simulink model "MOSSE_HDL_final"  (Simulink 8.3)
settings: Solver=FixedStepDiscrete  SolverMode=SingleTasking  StartTime=0.0  StopTime=30*640*360  RelTol=1e-3
InitFcn:
  | %% DSPBuilder Start
  | alt_dspbuilder_update_model(bdroot)
  | %% DSPBuilder End
  | param
StopFcn:
  | % r = rcount.Data(:,:);
  | % w = wcount.Data(:,:);
  | % d = dout.Data(:,:);
  | % ir = read.Data(:,:);
  | % iw = write.Data(:,:);
  | % z = double([ir iw d r w]');
  | %logic_analyzer
values from neighbouring files (symbols this model uses):
  Gau = [4035 -3983 3832 -3589 3269 -2890 2472 -2039 1612 -1211 854 -553 ... (4096 elements, 1x4096)]    [Gauss_coeff.mat]    (also in param.m = reshape(conj(Gau'), 1, 4096))
undefined symbols (not defined in the file or in its folder): gray, psr, source_1, source_2, State_Machine, State_Transition_Table1, window_hann
libraries: allblocks_alteradspbuilder2 x166, hdlsllib x24, hdldemolib x3, simulink x2, dspsigattribs x2, dspmtrx3 x2, visionsinks x1, visiontextngfix x1, dspvision x1
(part 2 of 4)

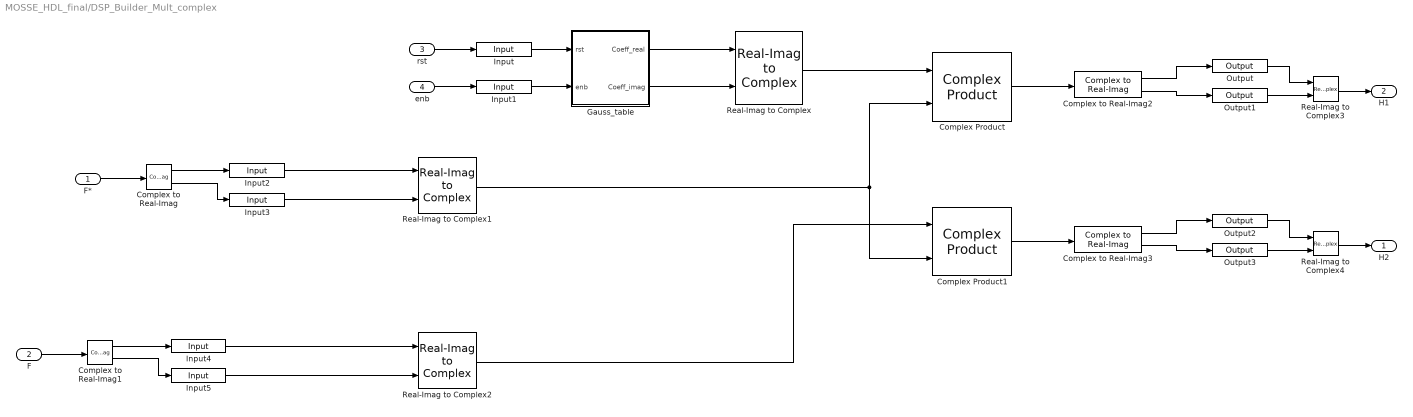
== system MOSSE_HDL_final/DSP_Builder_Mult_complex ==
  F* : Inport
  F : Inport  Port=2
  rst : Inport  Port=3
  enb : Inport  Port=4
  Complex Product : allblocks_alteradspbuilder2/Complex Product  BusType=Inferred  bwl=8  bwr=0  pipeline_register=Multiplier Only  pipeline_display=1  use_ena=off  use_aclr=off  UseDedicatedCircuitry=off  allowFloatingPointOverride=on  logOutputs=off  logFile=E:\Work\ComputerVision\ObjectTrack\MOSSE\autotrackigproject\Model\MOSSE_algorithm\MOSSE_simulink\tb_MOSSE_HDL_final\MOSSE%5FHDL%5Ffinal_DSP%5FBuilder%5FMult%5Fcomplex_Complex+Product.fixedpointlog
  Complex Product1 : allblocks_alteradspbuilder2/Complex Product  BusType=Inferred  bwl=8  bwr=0  pipeline_register=Multiplier Only  pipeline_display=1  use_ena=off  use_aclr=off  UseDedicatedCircuitry=off  allowFloatingPointOverride=on  logOutputs=off  logFile=E:\Work\ComputerVision\ObjectTrack\MOSSE\autotrackigproject\Model\MOSSE_algorithm\MOSSE_simulink\tb_MOSSE_HDL_final\MOSSE%5FHDL%5Ffinal_DSP%5FBuilder%5FMult%5Fcomplex_Complex+Product1.fixedpointlog
  Complex to Real-Imag : ComplexToRealImag
  Complex to Real-Imag1 : ComplexToRealImag
  Complex to Real-Imag2 : allblocks_alteradspbuilder2/Complex to Real-Imag  BusType=Signed Integer  bwl=32  bwr=0  pipeline_display=0  allowFloatingPointOverride=on  logOutputs=off  logFile=E:\Work\ComputerVision\ObjectTrack\MOSSE\autotrackigproject\Model\MOSSE_algorithm\MOSSE_simulink\tb_MOSSE_HDL_final\MOSSE%5FHDL%5Ffinal_DSP%5FBuilder%5FMult%5Fcomplex_Complex+to+Real-Imag2%3A%3Aoutput%5Freal.fixedpointlog,E:\Work\ComputerVision\ObjectTrack\MOSSE\autotrackigproject\Model\MOSSE_algorithm\MOSSE_simulink\tb_MOSSE_HDL_final\MOSSE%5FHDL%5Ffinal_DSP%5FBuilder%5FMult%5Fcomplex_Complex+to+Real-Imag2%3A%3Aoutput%5Fimag.fixedpointlog,
  Complex to Real-Imag3 : allblocks_alteradspbuilder2/Complex to Real-Imag  BusType=Signed Integer  bwl=32  bwr=0  pipeline_display=0  allowFloatingPointOverride=on  logOutputs=off  logFile=E:\Work\ComputerVision\ObjectTrack\MOSSE\autotrackigproject\Model\MOSSE_algorithm\MOSSE_simulink\tb_MOSSE_HDL_final\MOSSE%5FHDL%5Ffinal_DSP%5FBuilder%5FMult%5Fcomplex_Complex+to+Real-Imag3%3A%3Aoutput%5Freal.fixedpointlog,E:\Work\ComputerVision\ObjectTrack\MOSSE\autotrackigproject\Model\MOSSE_algorithm\MOSSE_simulink\tb_MOSSE_HDL_final\MOSSE%5FHDL%5Ffinal_DSP%5FBuilder%5FMult%5Fcomplex_Complex+to+Real-Imag3%3A%3Aoutput%5Fimag.fixedpointlog,
  Gauss_table : Subsystem
  Input : allblocks_alteradspbuilder2/Input  iofile=E:\Work\ComputerVision\ObjectTrack\MOSSE\autotrackigproject\Model\MOSSE_algorithm\MOSSE_simulink\tb_MOSSE_HDL_final\MOSSE%5FHDL%5Ffinal_DSP%5FBuilder%5FMult%5Fcomplex_Input.salt  BusType=Single Bit  bwl=8  bwr=0  SpecifyClock=off  PORTTYPE=Input  externalType=Inferred  allowFloatingPointOverride=on  logOutputs=off
  Input1 : allblocks_alteradspbuilder2/Input  iofile=E:\Work\ComputerVision\ObjectTrack\MOSSE\autotrackigproject\Model\MOSSE_algorithm\MOSSE_simulink\tb_MOSSE_HDL_final\MOSSE%5FHDL%5Ffinal_DSP%5FBuilder%5FMult%5Fcomplex_Input1.salt  BusType=Single Bit  bwl=8  bwr=0  SpecifyClock=off  PORTTYPE=Input  externalType=Inferred  allowFloatingPointOverride=on  logOutputs=off
  Input2 : allblocks_alteradspbuilder2/Input  iofile=E:\Work\ComputerVision\ObjectTrack\MOSSE\autotrackigproject\Model\MOSSE_algorithm\MOSSE_simulink\tb_MOSSE_HDL_final\MOSSE%5FHDL%5Ffinal_DSP%5FBuilder%5FMult%5Fcomplex_Input2.salt  BusType=Signed Integer  bwl=32  bwr=0  SpecifyClock=off  PORTTYPE=Input  externalType=Inferred  allowFloatingPointOverride=on  logOutputs=off
  Input3 : allblocks_alteradspbuilder2/Input  iofile=E:\Work\ComputerVision\ObjectTrack\MOSSE\autotrackigproject\Model\MOSSE_algorithm\MOSSE_simulink\tb_MOSSE_HDL_final\MOSSE%5FHDL%5Ffinal_DSP%5FBuilder%5FMult%5Fcomplex_Input3.salt  BusType=Signed Integer  bwl=32  bwr=0  SpecifyClock=off  PORTTYPE=Input  externalType=Inferred  allowFloatingPointOverride=on  logOutputs=off
  Input4 : allblocks_alteradspbuilder2/Input  iofile=E:\Work\ComputerVision\ObjectTrack\MOSSE\autotrackigproject\Model\MOSSE_algorithm\MOSSE_simulink\tb_MOSSE_HDL_final\MOSSE%5FHDL%5Ffinal_DSP%5FBuilder%5FMult%5Fcomplex_Input4.salt  BusType=Signed Integer  bwl=32  bwr=0  SpecifyClock=off  PORTTYPE=Input  externalType=Inferred  allowFloatingPointOverride=on  logOutputs=off
  Input5 : allblocks_alteradspbuilder2/Input  iofile=E:\Work\ComputerVision\ObjectTrack\MOSSE\autotrackigproject\Model\MOSSE_algorithm\MOSSE_simulink\tb_MOSSE_HDL_final\MOSSE%5FHDL%5Ffinal_DSP%5FBuilder%5FMult%5Fcomplex_Input5.salt  BusType=Signed Integer  bwl=32  bwr=0  SpecifyClock=off  PORTTYPE=Input  externalType=Inferred  allowFloatingPointOverride=on  logOutputs=off
  Output : allblocks_alteradspbuilder2/Output  iofile=E:\Work\ComputerVision\ObjectTrack\MOSSE\autotrackigproject\Model\MOSSE_algorithm\MOSSE_simulink\tb_MOSSE_HDL_final\MOSSE%5FHDL%5Ffinal_DSP%5FBuilder%5FMult%5Fcomplex_Output.capture  BusType=Signed Integer  bwl=32  bwr=0  externalType=Inferred  PORTTYPE=Output  allowFloatingPointOverride=on  logOutputs=off
  Output1 : allblocks_alteradspbuilder2/Output  iofile=E:\Work\ComputerVision\ObjectTrack\MOSSE\autotrackigproject\Model\MOSSE_algorithm\MOSSE_simulink\tb_MOSSE_HDL_final\MOSSE%5FHDL%5Ffinal_DSP%5FBuilder%5FMult%5Fcomplex_Output1.capture  BusType=Signed Integer  bwl=32  bwr=0  externalType=Simulink Fixed Point Type  PORTTYPE=Output  allowFloatingPointOverride=on  logOutputs=off
  Output2 : allblocks_alteradspbuilder2/Output  iofile=E:\Work\ComputerVision\ObjectTrack\MOSSE\autotrackigproject\Model\MOSSE_algorithm\MOSSE_simulink\tb_MOSSE_HDL_final\MOSSE%5FHDL%5Ffinal_DSP%5FBuilder%5FMult%5Fcomplex_Output2.capture  BusType=Signed Integer  bwl=32  bwr=0  externalType=Simulink Fixed Point Type  PORTTYPE=Output  allowFloatingPointOverride=on  logOutputs=off
  Output3 : allblocks_alteradspbuilder2/Output  iofile=E:\Work\ComputerVision\ObjectTrack\MOSSE\autotrackigproject\Model\MOSSE_algorithm\MOSSE_simulink\tb_MOSSE_HDL_final\MOSSE%5FHDL%5Ffinal_DSP%5FBuilder%5FMult%5Fcomplex_Output3.capture  BusType=Signed Integer  bwl=32  bwr=0  externalType=Simulink Fixed Point Type  PORTTYPE=Output  allowFloatingPointOverride=on  logOutputs=off
  Real-Imag to Complex3 : RealImagToComplex
  Real-Imag to Complex4 : RealImagToComplex
  Real-Imag to Complex : allblocks_alteradspbuilder2/Real-Imag to Complex  BusType=Signed Integer  bwl=16  bwr=0  pipeline_display=0  allowFloatingPointOverride=on  logOutputs=off  logFile=E:\Work\ComputerVision\ObjectTrack\MOSSE\autotrackigproject\Model\MOSSE_algorithm\MOSSE_simulink\tb_MOSSE_HDL_final\MOSSE%5FHDL%5Ffinal_DSP%5FBuilder%5FMult%5Fcomplex_Real-Imag+to+Complex.fixedpointlog
  Real-Imag to Complex1 : allblocks_alteradspbuilder2/Real-Imag to Complex  BusType=Signed Integer  bwl=32  bwr=0  pipeline_display=0  allowFloatingPointOverride=on  logOutputs=off  logFile=E:\Work\ComputerVision\ObjectTrack\MOSSE\autotrackigproject\Model\MOSSE_algorithm\MOSSE_simulink\tb_MOSSE_HDL_final\MOSSE%5FHDL%5Ffinal_DSP%5FBuilder%5FMult%5Fcomplex_Real-Imag+to+Complex1.fixedpointlog
  Real-Imag to Complex2 : allblocks_alteradspbuilder2/Real-Imag to Complex  BusType=Signed Integer  bwl=32  bwr=0  pipeline_display=0  allowFloatingPointOverride=on  logOutputs=off  logFile=E:\Work\ComputerVision\ObjectTrack\MOSSE\autotrackigproject\Model\MOSSE_algorithm\MOSSE_simulink\tb_MOSSE_HDL_final\MOSSE%5FHDL%5Ffinal_DSP%5FBuilder%5FMult%5Fcomplex_Real-Imag+to+Complex2.fixedpointlog
  H2 : Outport
  H1 : Outport  Port=2
  wires:
  Gauss_table/1(Coeff_real) -> Real-Imag to Complex/1
  Gauss_table/2(Coeff_imag) -> Real-Imag to Complex/2
  Real-Imag to Complex/1 -> Complex Product/1
  rst/1 -> Input/1
  Input/1 -> Gauss_table/1(rst)
  enb/1 -> Input1/1
  Input1/1 -> Gauss_table/2(enb)
  F*/1 -> Complex to Real-Imag/1
  F/1 -> Complex to Real-Imag1/1
  Complex to Real-Imag/1 -> Input2/1
  Complex to Real-Imag/2 -> Input3/1
  Complex to Real-Imag1/1 -> Input4/1
  Complex to Real-Imag1/2 -> Input5/1
  Input2/1 -> Real-Imag to Complex1/1
  Input3/1 -> Real-Imag to Complex1/2
  Input4/1 -> Real-Imag to Complex2/1
  Input5/1 -> Real-Imag to Complex2/2
  Real-Imag to Complex1/1 -> Complex Product1/2, Complex Product/2
  Real-Imag to Complex2/1 -> Complex Product1/1
  Complex Product/1 -> Complex to Real-Imag2/1
  Complex to Real-Imag2/2 -> Output1/1
  Complex to Real-Imag2/1 -> Output/1
  Real-Imag to Complex3/1 -> H1/1
  Output/1 -> Real-Imag to Complex3/1
  Output1/1 -> Real-Imag to Complex3/2
  Complex Product1/1 -> Complex to Real-Imag3/1
  Complex to Real-Imag3/2 -> Output3/1
  Complex to Real-Imag3/1 -> Output2/1
  Real-Imag to Complex4/1 -> H2/1
  Output2/1 -> Real-Imag to Complex4/1
  Output3/1 -> Real-Imag to Complex4/2

== system MOSSE_HDL_final/DSP_Builder_PSR ==
  max : Inport
  mean : Inport  Port=2
  tmp : Inport  Port=3
  psr_reset : Inport  Port=4
  Comparator : allblocks_alteradspbuilder2/Comparator  direction=a > b  pipeline_display=0  allowFloatingPointOverride=on  logOutputs=off  logFile=E:\Work\ComputerVision\ObjectTrack\MOSSE\autotrackigproject\Model\MOSSE_algorithm\MOSSE_simulink\tb_MOSSE_HDL_final\MOSSE%5FHDL%5Ffinal_DSP%5FBuilder%5FPSR_Comparator.fixedpointlog
  Constant : allblocks_alteradspbuilder2/Constant  mask_cst=PSR  BusType=Signed Integer  bwl=16  bwr=0  roundMode=Truncate  satMode=Wrap  SpecifyClock=off  allowFloatingPointOverride=on  logOutputs=off  logFile=E:\Work\ComputerVision\ObjectTrack\MOSSE\autotrackigproject\Model\MOSSE_algorithm\MOSSE_simulink\tb_MOSSE_HDL_final\MOSSE%5FHDL%5Ffinal_DSP%5FBuilder%5FPSR_Constant.fixedpointlog
  Data : allblocks_alteradspbuilder2/Input  iofile=E:\Work\ComputerVision\ObjectTrack\MOSSE\autotrackigproject\Model\MOSSE_algorithm\MOSSE_simulink\tb_MOSSE_HDL_final\MOSSE%5FHDL%5Ffinal_DSP%5FBuilder%5FPSR_Data.salt  BusType=Signed Integer  bwl=16  bwr=0  SpecifyClock=off  PORTTYPE=Input  externalType=Inferred  allowFloatingPointOverride=on  logOutputs=off
  Data1 : allblocks_alteradspbuilder2/Input  iofile=E:\Work\ComputerVision\ObjectTrack\MOSSE\autotrackigproject\Model\MOSSE_algorithm\MOSSE_simulink\tb_MOSSE_HDL_final\MOSSE%5FHDL%5Ffinal_DSP%5FBuilder%5FPSR_Data1.salt  BusType=Signed Integer  bwl=16  bwr=0  SpecifyClock=off  PORTTYPE=Input  externalType=Inferred  allowFloatingPointOverride=on  logOutputs=off
  Data2 : allblocks_alteradspbuilder2/Input  iofile=E:\Work\ComputerVision\ObjectTrack\MOSSE\autotrackigproject\Model\MOSSE_algorithm\MOSSE_simulink\tb_MOSSE_HDL_final\MOSSE%5FHDL%5Ffinal_DSP%5FBuilder%5FPSR_Data2.salt  BusType=Signed Integer  bwl=44  bwr=0  SpecifyClock=off  PORTTYPE=Input  externalType=Inferred  allowFloatingPointOverride=on  logOutputs=off
  Data3 : allblocks_alteradspbuilder2/Input  iofile=E:\Work\ComputerVision\ObjectTrack\MOSSE\autotrackigproject\Model\MOSSE_algorithm\MOSSE_simulink\tb_MOSSE_HDL_final\MOSSE%5FHDL%5Ffinal_DSP%5FBuilder%5FPSR_Data3.salt  BusType=Single Bit  bwl=44  bwr=0  SpecifyClock=off  PORTTYPE=Input  externalType=Inferred  allowFloatingPointOverride=on  logOutputs=off
  Delay : allblocks_alteradspbuilder2/Delay  pipeline=1  pipeline_display=1  ClockPhase=1  use_ena=off  use_sclr=off  allowFloatingPointOverride=on  logOutputs=off  logFile=E:\Work\ComputerVision\ObjectTrack\MOSSE\autotrackigproject\Model\MOSSE_algorithm\MOSSE_simulink\tb_MOSSE_HDL_final\MOSSE%5FHDL%5Ffinal_DSP%5FBuilder%5FPSR_Delay.fixedpointlog  use_init=off  reset_value=1
  Delay1 : allblocks_alteradspbuilder2/Delay  pipeline=1  pipeline_display=1  ClockPhase=1  use_ena=off  use_sclr=off  allowFloatingPointOverride=on  logOutputs=off  logFile=E:\Work\ComputerVision\ObjectTrack\MOSSE\autotrackigproject\Model\MOSSE_algorithm\MOSSE_simulink\tb_MOSSE_HDL_final\MOSSE%5FHDL%5Ffinal_DSP%5FBuilder%5FPSR_Delay1.fixedpointlog  use_init=off  reset_value=1
  Delay2 : allblocks_alteradspbuilder2/Delay  pipeline=1  pipeline_display=1  ClockPhase=1  use_ena=off  use_sclr=on  allowFloatingPointOverride=on  logOutputs=off  logFile=E:\Work\ComputerVision\ObjectTrack\MOSSE\autotrackigproject\Model\MOSSE_algorithm\MOSSE_simulink\tb_MOSSE_HDL_final\MOSSE%5FHDL%5Ffinal_DSP%5FBuilder%5FPSR_Delay2.fixedpointlog  use_init=off  reset_value=1
  Divider : allblocks_alteradspbuilder2/Divider  BusType=Signed Integer  bwl=32  bwr=0  pipeline=5  pipeline_display=5  use_ena=off  use_aclr=off
  Pipelined Adder : allblocks_alteradspbuilder2/Pipelined Adder  BusType=Signed Integer  bwl=32  bwr=0  pipeline=0  pipeline_display=0  AddSubDirection=SUB  use_cin=off  use_ovl=off  use_addsub=off  use_ena=off  use_aclr=off  or_aclr_inputs=on
  Square Root : allblocks_alteradspbuilder2/Square Root  BusType=Unsigned Integer  bwl=44  bwr=0  pipeline=2  pipeline_display=2  use_remain=off  use_ena=off  use_aclr=off
  Terminator : Terminator
  max_Num : allblocks_alteradspbuilder2/Output  iofile=E:\Work\ComputerVision\ObjectTrack\MOSSE\autotrackigproject\Model\MOSSE_algorithm\MOSSE_simulink\tb_MOSSE_HDL_final\MOSSE%5FHDL%5Ffinal_DSP%5FBuilder%5FPSR_max%5FNum.capture  BusType=Signed Integer  bwl=16  bwr=0  externalType=Simulink Fixed Point Type  PORTTYPE=Output  allowFloatingPointOverride=on  logOutputs=off
  max_Num1 : allblocks_alteradspbuilder2/Output  iofile=E:\Work\ComputerVision\ObjectTrack\MOSSE\autotrackigproject\Model\MOSSE_algorithm\MOSSE_simulink\tb_MOSSE_HDL_final\MOSSE%5FHDL%5Ffinal_DSP%5FBuilder%5FPSR_max%5FNum1.capture  BusType=Single Bit  bwl=16  bwr=0  externalType=Simulink Fixed Point Type  PORTTYPE=Output  allowFloatingPointOverride=on  logOutputs=off
  psr : Outport
  psr_check : Outport  Port=2
  wires:
  Pipelined Adder/1 -> Delay/1
  Square Root/1 -> Delay1/1
  Divider/1 -> Delay2/1
  Data/1 -> Pipelined Adder/1
  Data1/1 -> Pipelined Adder/2
  Data2/1 -> Square Root/1
  tmp/1 -> Data2/1
  Divider/2 -> Terminator/1
  mean/1 -> Data1/1
  max/1 -> Data/1
  max_Num/1 -> psr/1
  Delay1/1 -> Divider/2
  Delay/1 -> Divider/1
  Delay2/1 -> Comparator/1, max_Num/1
  Data3/1 -> Delay2/2
  psr_reset/1 -> Data3/1
  Constant/1 -> Comparator/2
  Comparator/1 -> max_Num1/1
  max_Num1/1 -> psr_check/1

== system MOSSE_HDL_final/DSP_Builder_Smoothing_Window ==
  ipixel : Inport
  rst : Inport  Port=2
  enb : Inport  Port=3
  Barrel Shifter : allblocks_alteradspbuilder2/Barrel Shifter  BusType=Unsigned Integer  bwl=16  bwr=8  pipeline=off  infer_distance=off  distance_length=4  ShiftDirection=Shift right  use_ena=off  use_aclr=off  UseDedicatedCircuitry=off  pipeline_display=0  allowFloatingPointOverride=on  logOutputs=off  logFile=E:\Work\ComputerVision\ObjectTrack\MOSSE\autotrackigproject\Model\MOSSE_algorithm\MOSSE_simulink\tb_MOSSE_HDL_final\MOSSE%5FHDL%5Ffinal_DSP%5FBuilder%5FSmoothing%5FWindow_Barrel+Shifter.fixedpointlog
  Constant : allblocks_alteradspbuilder2/Constant  mask_cst=8  BusType=Unsigned Integer  bwl=4  bwr=0  roundMode=Truncate  satMode=Wrap  SpecifyClock=off  allowFloatingPointOverride=on  logOutputs=off  logFile=E:\Work\ComputerVision\ObjectTrack\MOSSE\autotrackigproject\Model\MOSSE_algorithm\MOSSE_simulink\tb_MOSSE_HDL_final\MOSSE%5FHDL%5Ffinal_DSP%5FBuilder%5FSmoothing%5FWindow_Constant.fixedpointlog
  Counter : allblocks_alteradspbuilder2/Counter  BusType=Unsigned Integer  bwl=12  bwr=0  use_modulo=off  modulo=255  SpecifyClock=off  direction=Increment  use_sload=off  use_sset=off  svalue=1  use_clk_ena=off  use_ena=on  use_sclr=on  pipeline_display=1
  Input : allblocks_alteradspbuilder2/Input  iofile=E:\Work\ComputerVision\ObjectTrack\MOSSE\autotrackigproject\Model\MOSSE_algorithm\MOSSE_simulink\tb_MOSSE_HDL_final\MOSSE%5FHDL%5Ffinal_DSP%5FBuilder%5FSmoothing%5FWindow_Input.salt  BusType=Unsigned Integer  bwl=8  bwr=0  SpecifyClock=off  PORTTYPE=Input  externalType=Inferred  allowFloatingPointOverride=on  logOutputs=off
  Input1 : allblocks_alteradspbuilder2/Input  iofile=E:\Work\ComputerVision\ObjectTrack\MOSSE\autotrackigproject\Model\MOSSE_algorithm\MOSSE_simulink\tb_MOSSE_HDL_final\MOSSE%5FHDL%5Ffinal_DSP%5FBuilder%5FSmoothing%5FWindow_Input1.salt  BusType=Single Bit  bwl=8  bwr=0  SpecifyClock=off  PORTTYPE=Input  externalType=Inferred  allowFloatingPointOverride=on  logOutputs=off
  Input2 : allblocks_alteradspbuilder2/Input  iofile=E:\Work\ComputerVision\ObjectTrack\MOSSE\autotrackigproject\Model\MOSSE_algorithm\MOSSE_simulink\tb_MOSSE_HDL_final\MOSSE%5FHDL%5Ffinal_DSP%5FBuilder%5FSmoothing%5FWindow_Input2.salt  BusType=Single Bit  bwl=8  bwr=0  SpecifyClock=off  PORTTYPE=Input  externalType=Inferred  allowFloatingPointOverride=on  logOutputs=off
  Output : allblocks_alteradspbuilder2/Output  iofile=E:\Work\ComputerVision\ObjectTrack\MOSSE\autotrackigproject\Model\MOSSE_algorithm\MOSSE_simulink\tb_MOSSE_HDL_final\MOSSE%5FHDL%5Ffinal_DSP%5FBuilder%5FSmoothing%5FWindow_Output.capture  BusType=Unsigned Integer  bwl=8  bwr=0  externalType=Simulink Fixed Point Type  PORTTYPE=Output  allowFloatingPointOverride=on  logOutputs=off
  Product : allblocks_alteradspbuilder2/Product  BusType=Unsigned Integer  bwl=8  bwr=0  pipeline=1  pipeline_display=1  phase_selection=1  use_ena=off  use_aclr=off  UseLPM=off  UseDedicatedCircuitry=off  allowFloatingPointOverride=on  logOutputs=off  logFile=E:\Work\ComputerVision\ObjectTrack\MOSSE\autotrackigproject\Model\MOSSE_algorithm\MOSSE_simulink\tb_MOSSE_HDL_final\MOSSE%5FHDL%5Ffinal_DSP%5FBuilder%5FSmoothing%5FWindow_Product.fixedpointlog
  ROM : allblocks_alteradspbuilder2/ROM  numwords=4096  BusType=Unsigned Integer  bwl=8  bwr=0  memory_type=AUTO  ram_type=ROM  initialization=From MATLAB array  init_file=input.hex  init_array=reshape(window_hann', 1, 4096)  register_outputs=off  use_ena=off  ClockPhase=1  pipeline_display=1  allowFloatingPointOverride=on  logOutputs=off  logFile=E:\Work\ComputerVision\ObjectTrack\MOSSE\autotrackigproject\Model\MOSSE_algorithm\MOSSE_simulink\tb_MOSSE_HDL_final\MOSSE%5FHDL%5Ffinal_DSP%5FBuilder%5FSmoothing%5FWindow_ROM.fixedpointlog  enable_runtime_mod=off  instance_name=AAAA
  opixel : Outport
  wires:
  enb/1 -> Input1/1
  rst/1 -> Input2/1
  Counter/1 -> ROM/1
  ipixel/1 -> Input/1
  Input/1 -> Product/1
  Output/1 -> opixel/1
  Input1/1 -> Counter/1
  Input2/1 -> Counter/2
  Barrel Shifter/1 -> Output/1
  Product/1 -> Barrel Shifter/1
  Constant/1 -> Barrel Shifter/2
  ROM/1 -> Product/2

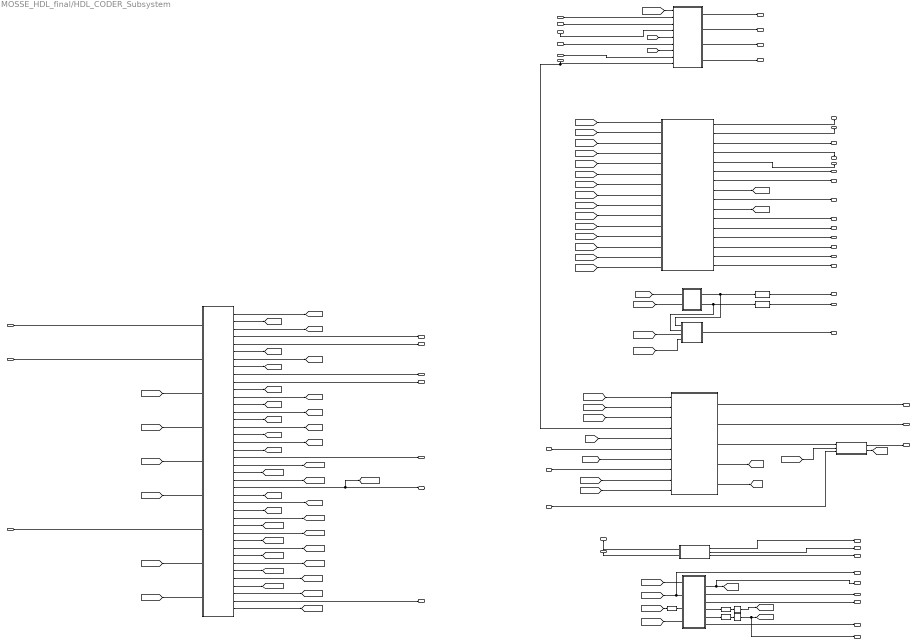
== system MOSSE_HDL_final/HDL_CODER_Subsystem ==
  G : Inport
  F : Inport  Port=2
  "H2 " : Inport  Port=3
  iPixel_image : Inport  Port=4
  H1_alfa : Inport  Port=5
  H2_alfa : Inport  Port=6
  H1 : Inport  Port=7
  H1_p : Inport  Port=8
  H2_p : Inport  Port=9
  In12 : Inport  Port=10
  iCorr_data : Inport  Port=11
  enable_Tracking : Inport  Port=12
  psr_check : Inport  Port=13
  enable_write : Inport  Port=14
  Comp_Shift_code_Subsys : Subsystem
  Complex_2_real_imag : Subsystem
  Data Type Conversion : DataTypeConversion  OutDataTypeStr=int8
  Data Type Conversion1 : DataTypeConversion  OutDataTypeStr=int8
  Data Type Conversion2 : DataTypeConversion  OutDataTypeStr=int16
  Data Type Conversion20 : DataTypeConversion  OutDataTypeStr=boolean
  Data Type Conversion21 : DataTypeConversion  OutDataTypeStr=boolean
  Delay2 : Delay  DelayLength=1  InitialCondition=0
  Delay3 : Delay  DelayLength=3  InitialCondition=0
  FFT2D_System : Subsystem
  IFFT_MUX : Subsystem
  Main_State_Machine : Subsystem
  Memory_Counter_Subsys : Subsystem
  Mux_system : Subsystem
  SM_memory : Subsystem
  psr_code_subsys : Subsystem
  oH2 : Outport
  wr_addr_H1_H2 : Outport  Port=2
  we_H1_H2 : Outport  Port=3
  wr_addr_G_F : Outport  Port=4
  we_G_F : Outport  Port=5
  addr_in_im : Outport  Port=6
  rd_addr_H1_H2 : Outport  Port=7
  rd_addr_G_F : Outport  Port=8
  we_m : Outport  Port=9
  oH1 : Outport  Port=10
  oData1 : Outport  Port=11
  Real_H1 : Outport  Port=12
  Real_H2 : Outport  Port=13
  Imag_H1 : Outport  Port=14
  oData2 : Outport  Port=15
  oF* : Outport  Port=16
  wr_addr_H : Outport  Port=17
  oF : Outport  Port=18
  we_H : Outport  Port=19
  rd_addr_H : Outport  Port=20
  RAM_data : Outport  Port=21
  wr_addr_RAM_IFFT : Outport  Port=22
  we_RAM_IFFT : Outport  Port=23
  addr_memory_128x128 : Outport  Port=24
  rst_win : Outport  Port=25
  enb_win : Outport  Port=26
  rst_gauss : Outport  Port=27
  enb_gauss : Outport  Port=28
  div_complex : Outport  Port=29
  comp_shift_finish : Outport  Port=30
  to_workspace_enb : Outport  Port=31
  rd_addr_RAM_IFFT : Outport  Port=32
  Dx : Outport  Port=33
  Dy : Outport  Port=34
  max_val : Outport  Port=35
  mean_val : Outport  Port=36
  tmp_val : Outport  Port=37
  psr_reset : Outport  Port=38
  psr_finish : Outport  Port=39
  max_index : Outport  Port=40
  wires:
  [mem_count_clear] -> Memory_Counter_Subsys/3(clear)
  [mem_count_en] -> Memory_Counter_Subsys/4(en)
  Memory_Counter_Subsys/1(addr) -> addr_memory_128x128/1
  [img_finish] -> Main_State_Machine/3(img_finish)
  [end_fft] -> Main_State_Machine/4(end_fft)
  [data_ready] -> Main_State_Machine/5(data_ready)
  [read_H_finish] -> Main_State_Machine/6(read_H_finish)
  psr_check/1 -> Main_State_Machine/7(psr_check)
  [psr_finish] -> Main_State_Machine/8(psr_finish)
  [psr_mean_finish] -> Main_State_Machine/9(psr_mean_finish)
  Main_State_Machine/1(en_img) -> [en_img]
  Main_State_Machine/2(read_img) -> [read_img]
  Main_State_Machine/3(write_img) -> [write_img]
  Main_State_Machine/4(rst_win) -> rst_win/1
  Main_State_Machine/5(enb_win) -> enb_win/1
  Main_State_Machine/6(mux_fft_ifft) -> [mux_fft_ifft]
  Main_State_Machine/7(start_fft_ifft) -> [start_fft_ifft]
  Main_State_Machine/8(enb_fft_ifft) -> [enb_fft_ifft]
  Main_State_Machine/9(rst_gauss) -> rst_gauss/1
  Main_State_Machine/10(enb_gauss) -> enb_gauss/1
  Main_State_Machine/11(mux_mult) -> [mux_mult]
  Main_State_Machine/12(en_m_ram_g) -> [en_m_ram_g]
  Main_State_Machine/13(read_g) -> [read_g]
  Main_State_Machine/14(write_g) -> [write_g]
  Main_State_Machine/15(enb_H_ram) -> [enb_H_ram]
  Main_State_Machine/16(read_H_ram) -> [read_H_ram]
  Main_State_Machine/17(write_H_ram) -> [write_H_ram]
  Main_State_Machine/18(mux_H2) -> [mux_H2]
  Main_State_Machine/19(mux_H1) -> [mux_H1]
  Main_State_Machine/20(div_complex_aclr) -> div_complex/1
  Main_State_Machine/21(enb_div_ram) -> [enb_div_ram]
  Main_State_Machine/22(read_div_ram) -> [read_div_ram]
  Main_State_Machine/23(write_div_ram) -> [write_div_ram]
  Main_State_Machine/25(en_r) -> [en_r]
  Main_State_Machine/26(read_r) -> [read_r]
  Main_State_Machine/27(write_r) -> [write_r]
  Main_State_Machine/28(en_ifft_res) -> [en_ifft_res]
  Main_State_Machine/29(read_ifft_res) -> [read_ifft_res]
  Main_State_Machine/30(write_ifft_res) -> [write_ifft_res]
  Main_State_Machine/31(enb_psr) -> [enb_psr]
  Main_State_Machine/32(comp_shift_iaclr) -> [comp_shift_iaclr]
  Main_State_Machine/33(mem_count_clear) -> [mem_count_clear]
  Main_State_Machine/34(mem_count_en) -> [mem_count_en]
  Main_State_Machine/35(psr_reset) -> [psr_reset]
  Main_State_Machine/36(ifft_res_mult) -> [ifft_res_mult]
  Main_State_Machine/37(g_out_contr) -> [g_out_contr]
  Main_State_Machine/38(to_workspace_write) -> [to_workspace_write]
  enable_write/1 -> Main_State_Machine/2(enable_write)
  enable_Tracking/1 -> Main_State_Machine/1(enable_in)
  IFFT_MUX/1(RAM_data) -> RAM_data/1
  [ifft_res_mult] -> IFFT_MUX/2(Mux)
  In12/1 -> IFFT_MUX/3(IFFT_res1)
  IFFT_MUX/2(oData) -> [oData]
  Complex_2_real_imag/1(Real_H1) -> Real_H1/1
  Complex_2_real_imag/2(Real_H2) -> Real_H2/1
  Complex_2_real_imag/3(Imag_H1) -> Imag_H1/1
  [g_out_contr] -> Mux_system/1(iMux_Mult)
  G/1 -> Mux_system/2(iData1)
  F/1 -> Mux_system/3(iData2)
  [mux_H1] -> Mux_system/5(iMux_H1)
  [mux_H2] -> Mux_system/7(iMux_H2)
  H1_alfa/1 -> Mux_system/6(iH1_2)
  H2_alfa/1 -> Mux_system/8(iH2_2)
  Mux_system/1(H2) -> oH2/1
  [write_r] -> FFT2D_System/3(write_R)
  Mux_system/2(H1) -> oH1/1
  Mux_system/3(oData1) -> oData1/1
  Mux_system/4(oData2) -> oData2/1
  [en_r] -> FFT2D_System/1(en_R)
  [read_r] -> FFT2D_System/2(read_R)
  [mux_mult] -> FFT2D_System/5(iMux_mult)
  iCorr_data/1 -> FFT2D_System/6(Corr_Data)
  [mux_fft_ifft] -> FFT2D_System/7(Mux)
  iPixel_image/1 -> FFT2D_System/8(image)
  [start_fft_ifft] -> FFT2D_System/9(Start)
  [enb_fft_ifft] -> FFT2D_System/10(Enb)
  FFT2D_System/1(F*) -> oF*/1
  FFT2D_System/2(F) -> oF/1
  FFT2D_System/3(IFFT_res) -> IFFT_MUX/1(IFFT_res)
  FFT2D_System/5(end) -> [end_fft]
  FFT2D_System/4(data_ready) -> [data_ready]
  SM_memory/1(wr_addr_G_F) -> wr_addr_G_F/1
  SM_memory/2(we_G_F) -> we_G_F/1
  SM_memory/5(rd_addr_G_F) -> rd_addr_G_F/1
  SM_memory/4(we_H1_H2) -> we_H1_H2/1
  SM_memory/6(rd_addr_H1_H2) -> rd_addr_H1_H2/1
  SM_memory/3(wr_addr_H1_H2) -> wr_addr_H1_H2/1
  [enb_H_ram] -> SM_memory/1(en_H1_H2)
  [en_m_ram_g] -> SM_memory/2(en_G_F)
  [read_H_ram] -> SM_memory/3(rd_H1_H2)
  [read_g] -> SM_memory/4(rd_G_F)
  [write_H_ram] -> SM_memory/5(wr_H1_H2)
  [write_g] -> SM_memory/6(wr_G_F)
  [en_img] -> SM_memory/7(en_im_in)
  [read_img] -> SM_memory/8(rd_im_in)
  [write_img] -> SM_memory/9(wr_im_in)
  [enb_div_ram] -> SM_memory/10(en_H)
  [read_div_ram] -> SM_memory/11(rd_H)
  [write_div_ram] -> SM_memory/12(wr_H)
  [en_ifft_res] -> SM_memory/13(en_RAM_IFFT)
  [read_ifft_res] -> SM_memory/14(rd_RAM_IFFT)
  [write_ifft_res] -> SM_memory/15(wr_RAM_IFFT)
  SM_memory/7(addr_in_im) -> addr_in_im/1
  SM_memory/9(we_m) -> we_m/1
  SM_memory/8(oflag_H1_H2) -> [read_H_finish]
  SM_memory/11(wr_addr_H) -> wr_addr_H/1
  SM_memory/10(oflag) -> [img_finish]
  SM_memory/12(we_H) -> we_H/1
  SM_memory/13(rd_addr_H) -> rd_addr_H/1
  SM_memory/15(we_RAM_IFFT) -> we_RAM_IFFT/1
  SM_memory/14(wr_addr_RAM_IFFT) -> wr_addr_RAM_IFFT/1
  H2_p/1 -> Complex_2_real_imag/2(H2)
  H1/1 -> Mux_system/4(iH1_1)
  H1_p/1 -> Complex_2_real_imag/1(H1)
  "H2 "/1 -> FFT2D_System/4(iData), Mux_system/9(iH2_1)
  Main_State_Machine/39(comp_shift_finish) -> comp_shift_finish/1
  Main_State_Machine/24(to_workspace_enb) -> [to_workspace_enb], to_workspace_enb/1
  Main_State_Machine/40(count_std_enb) -> [count_std_enb]
  SM_memory/16(rd_addr_RAM_IFFT) -> rd_addr_RAM_IFFT/1
  [max_index] -> Comp_Shift_code_Subsys/1(Max_num)
  [comp_shift_iaclr] -> Comp_Shift_code_Subsys/2(iaclr)
  Comp_Shift_code_Subsys/1(dx) -> Memory_Counter_Subsys/1(dx), Data Type Conversion1/1
  Comp_Shift_code_Subsys/2(dy) -> Memory_Counter_Subsys/2(dy), Data Type Conversion/1
  Data Type Conversion1/1 -> Dx/1
  Data Type Conversion/1 -> Dy/1
  [enb_psr] -> psr_code_subsys/1(enb)
  [psr_reset] -> psr_reset/1, psr_code_subsys/2(rst)
  [oData] -> Data Type Conversion2/1
  [count_std_enb] -> psr_code_subsys/4(count_std_enb)
  Data Type Conversion2/1 -> psr_code_subsys/3(idata)
  Data Type Conversion20/1 -> Delay2/1
  Data Type Conversion21/1 -> Delay3/1
  psr_code_subsys/5(mean_finish) -> Data Type Conversion20/1
  psr_code_subsys/6(psr_finish) -> Data Type Conversion21/1
  psr_code_subsys/2(max_index) -> max_index/1, [max_index]
  Delay3/1 -> psr_finish/1, [psr_finish]
  Delay2/1 -> [psr_mean_finish]
  psr_code_subsys/3(max_value) -> max_val/1
  psr_code_subsys/4(mean_value) -> mean_val/1
  psr_code_subsys/7(std_value) -> tmp_val/1

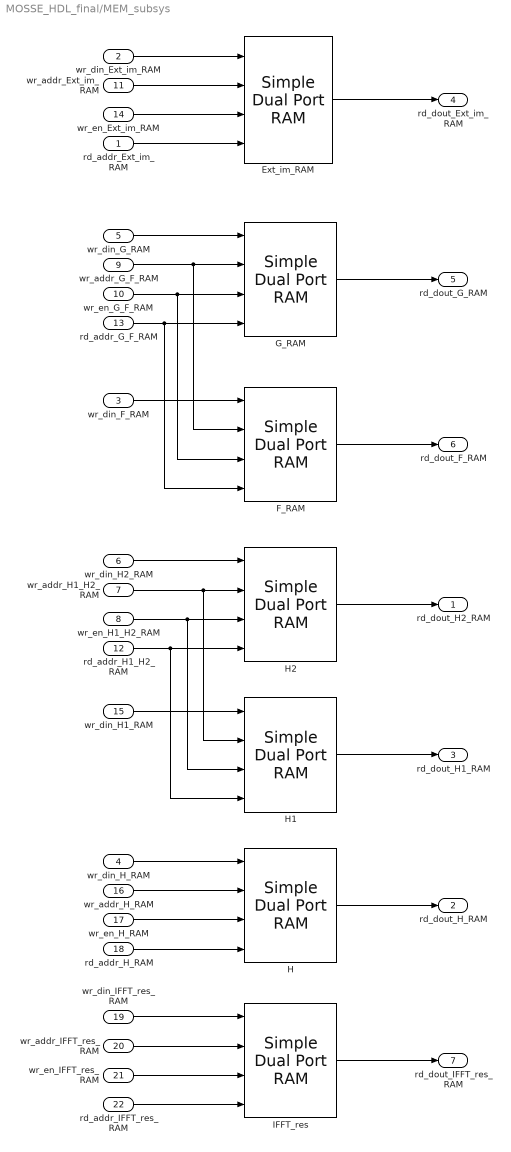
== system MOSSE_HDL_final/MEM_subsys ==
  rd_addr_Ext_im_RAM : Inport
  wr_din_Ext_im_RAM : Inport  Port=2
  wr_din_F_RAM : Inport  Port=3
  wr_din_H_RAM : Inport  Port=4
  wr_din_G_RAM : Inport  Port=5
  wr_din_H2_RAM : Inport  Port=6
  wr_addr_H1_H2_RAM : Inport  Port=7
  wr_en_H1_H2_RAM : Inport  Port=8
  wr_addr_G_F_RAM : Inport  Port=9
  wr_en_G_F_RAM : Inport  Port=10
  wr_addr_Ext_im_RAM : Inport  Port=11
  rd_addr_H1_H2_RAM : Inport  Port=12
  rd_addr_G_F_RAM : Inport  Port=13
  wr_en_Ext_im_RAM : Inport  Port=14
  wr_din_H1_RAM : Inport  Port=15
  wr_addr_H_RAM : Inport  Port=16
  wr_en_H_RAM : Inport  Port=17
  rd_addr_H_RAM : Inport  Port=18
  wr_din_IFFT_res_RAM : Inport  Port=19
  wr_addr_IFFT_res_RAM : Inport  Port=20
  wr_en_IFFT_res_RAM : Inport  Port=21
  rd_addr_IFFT_res_RAM : Inport  Port=22
  Ext_im_RAM : hdlsllib/HDL Operations/Simple Dual Port RAM  ram_size=14
  F_RAM : hdlsllib/HDL Operations/Simple Dual Port RAM  ram_size=12
  G_RAM : hdlsllib/HDL Operations/Simple Dual Port RAM  ram_size=12
  H : hdlsllib/HDL Operations/Simple Dual Port RAM  ram_size=12
  H1 : hdlsllib/HDL Operations/Simple Dual Port RAM  ram_size=12
  H2 : hdlsllib/HDL Operations/Simple Dual Port RAM  ram_size=12
  IFFT_res : hdlsllib/HDL Operations/Simple Dual Port RAM  ram_size=12
  rd_dout_H2_RAM : Outport
  rd_dout_H_RAM : Outport  Port=2
  rd_dout_H1_RAM : Outport  Port=3
  rd_dout_Ext_im_RAM : Outport  Port=4
  rd_dout_G_RAM : Outport  Port=5
  rd_dout_F_RAM : Outport  Port=6
  rd_dout_IFFT_res_RAM : Outport  Port=7
  wires:
  wr_din_Ext_im_RAM/1 -> Ext_im_RAM/1
  wr_addr_Ext_im_RAM/1 -> Ext_im_RAM/2
  wr_en_Ext_im_RAM/1 -> Ext_im_RAM/3
  rd_addr_Ext_im_RAM/1 -> Ext_im_RAM/4
  Ext_im_RAM/1 -> rd_dout_Ext_im_RAM/1
  wr_din_G_RAM/1 -> G_RAM/1
  G_RAM/1 -> rd_dout_G_RAM/1
  wr_din_F_RAM/1 -> F_RAM/1
  F_RAM/1 -> rd_dout_F_RAM/1
  rd_addr_G_F_RAM/1 -> F_RAM/4, G_RAM/4
  wr_en_G_F_RAM/1 -> F_RAM/3, G_RAM/3
  wr_addr_G_F_RAM/1 -> F_RAM/2, G_RAM/2
  H2/1 -> rd_dout_H2_RAM/1
  H1/1 -> rd_dout_H1_RAM/1
  wr_din_H2_RAM/1 -> H2/1
  wr_din_H1_RAM/1 -> H1/1
  rd_addr_H1_H2_RAM/1 -> H1/4, H2/4
  wr_en_H1_H2_RAM/1 -> H1/3, H2/3
  wr_addr_H1_H2_RAM/1 -> H1/2, H2/2
  H/1 -> rd_dout_H_RAM/1
  rd_addr_H_RAM/1 -> H/4
  wr_en_H_RAM/1 -> H/3
  wr_addr_H_RAM/1 -> H/2
  wr_din_H_RAM/1 -> H/1
  IFFT_res/1 -> rd_dout_IFFT_res_RAM/1
  wr_din_IFFT_res_RAM/1 -> IFFT_res/1
  wr_addr_IFFT_res_RAM/1 -> IFFT_res/2
  wr_en_IFFT_res_RAM/1 -> IFFT_res/3
  rd_addr_IFFT_res_RAM/1 -> IFFT_res/4

== system MOSSE_HDL_final/Source ==
  note: Тестовые последовательности
  source_control : Inport
  source_enb : Inport  Port=2
  source_count_rst : Inport  Port=3
  source_count_enb : Inport  Port=4
  source1_enb : Inport  Port=5
  ADDR_iPix1 : hdldemolib/HDL Counter  CountType=Free running  CountInit=0  CountStep=1  CountMax=100  CountFromType=Initial value  CountFrom=0  CountResetPort=on  CountLoadPort=off  CountEnbPort=on  CountDirPort=off  CountDataType=Unsigned  CountWordLen=32  CountFracLen=0  CountSampTime=1
  FFT/IFTT Mux1 : MultiPortSwitch  DataPortOrder=Zero-based contiguous  Inputs=2  zeroidx=on  OutDataTypeStr=fixdt(1,24,0)  SampleTime=1
  State Transition Table : State Transition Table  Commented=on  TreatAsAtomicUnit=on
  source_1 : Subsystem
  source_2 : Subsystem
  Out : Outport
  address : Outport  Port=2
  wires:
  ADDR_iPix1/1 -> address/1, State Transition Table/1(address), source_2/1(In1), source_1/1(In1)
  source_enb/1 -> source_1/Enable
  source1_enb/1 -> source_2/Enable
  source_count_enb/1 -> ADDR_iPix1/2
  FFT/IFTT Mux1/1 -> Out/1
  source_count_rst/1 -> ADDR_iPix1/1
  source_1/1(Out1) -> FFT/IFTT Mux1/2
  source_control/1 -> FFT/IFTT Mux1/1
  source_2/1(Out1) -> FFT/IFTT Mux1/3
  State Transition Table/1(enable_write) -> ?

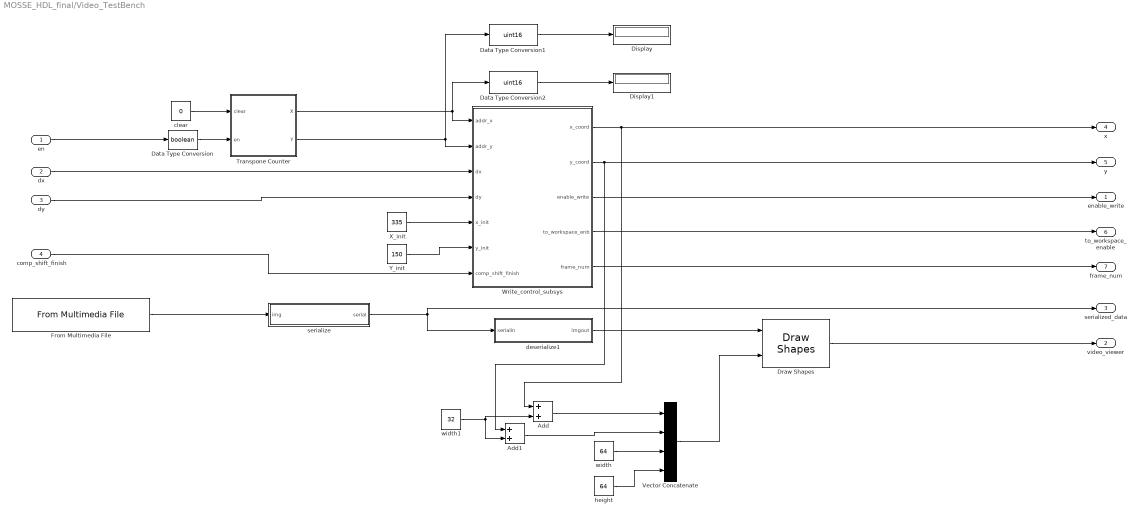
== system MOSSE_HDL_final/Video_TestBench ==
  en : Inport
  dx : Inport  Port=2
  dy : Inport  Port=3
  comp_shift_finish : Inport  Port=4
  Add : Sum  AccumDataTypeStr=uint16
  Add1 : Sum  AccumDataTypeStr=uint16
  Data Type Conversion : DataTypeConversion  OutDataTypeStr=boolean
  Data Type Conversion1 : DataTypeConversion  OutDataTypeStr=uint16
  Data Type Conversion2 : DataTypeConversion  OutDataTypeStr=uint16
  Display : Display
  Display1 : Display
  Draw Shapes : visiontextngfix/Draw Shapes  shape=Rectangles  fill=off  lineWidth=1  fillClrSource=Specify via dialog  display=User-specified value  intensity=200  color=[255]  opacity=0.6  viewport=Entire image  antialiasing=off  inType=Obsolete  imagePorts=One multidimensional signal  prodOutputMode=Binary point scaling  prodOutputWordLength=32  prodOutputFracLength=14  memoryMode=Specify word length  memoryWordLength=16  memoryFracLength=15  roundingMode=Floor  overflowMode=off
  From Multimedia File : dspvision/From Multimedia File  inputFilename=E:\Work\ComputerVision\ObjectTrack\MOSSE\autotrackigproject\Model\MOSSE_algorithm\MOSSE_simulink\klt_algorithm_robustness_640x360.avi  loop=on  numPlays=inf  outputStreams=Video only  videoDataType=uint8  audioDataType=int16  inheritSampleTime=off  userDefinedSampleTime=640*360  noAudioOutput=off  isIntensityVideo=off  fourcc=Intensity  colorVideoFormat=One multidimensional signal  outputEOF=off  dataOrg=Column-major  audioFrameSize=1024  computeAudioFrameSize=off  outSamplingMode=Sample based
  Transpone Counter : MATLAB Function
  Vector Concatenate : Concatenate  NumInputs=4
  Write_control_subsys : Subsystem
  X_init : Constant  Value=335  OutDataTypeStr=uint16
  Y_init : Constant  Value=150  OutDataTypeStr=uint16
  clear : Constant  Value=0  OutDataTypeStr=boolean
  deserialize1 : Subsystem
  height : Constant  Value=64  OutDataTypeStr=uint16
  serialize : Subsystem
  width : Constant  Value=64  OutDataTypeStr=uint16
  width1 : Constant  Value=32  OutDataTypeStr=uint16
  enable_write : Outport
  video_viewer : Outport  Port=2
  serialized_data : Outport  Port=3
  x : Outport  Port=4
  y : Outport  Port=5
  to_workspace_enable : Outport  Port=6
  frame_num : Outport  Port=7
  wires:
  From Multimedia File/1 -> serialize/1(img)
  deserialize1/1(imgout) -> Draw Shapes/1
  Transpone Counter/2(Y) -> Write_control_subsys/2(addr_y), Data Type Conversion1/1
  Transpone Counter/1(X) -> Write_control_subsys/1(addr_x), Data Type Conversion2/1
  Data Type Conversion/1 -> Transpone Counter/2(en)
  clear/1 -> Transpone Counter/1(clear)
  en/1 -> Data Type Conversion/1
  Draw Shapes/1 -> video_viewer/1
  width/1 -> Vector Concatenate/3
  height/1 -> Vector Concatenate/4
  Vector Concatenate/1 -> Draw Shapes/2
  Add1/1 -> Vector Concatenate/2
  Add/1 -> Vector Concatenate/1
  Data Type Conversion1/1 -> Display/1
  Data Type Conversion2/1 -> Display1/1
  width1/1 -> Add/2, Add1/2
  Write_control_subsys/1(x_coord) -> Add/1, x/1
  Write_control_subsys/2(y_coord) -> Add1/1, y/1
  dx/1 -> Write_control_subsys/3(dx)
  dy/1 -> Write_control_subsys/4(dy)
  Y_init/1 -> Write_control_subsys/6(y_init)
  comp_shift_finish/1 -> Write_control_subsys/7(comp_shift_finish)
  Write_control_subsys/3(enable_write) -> enable_write/1
  Write_control_subsys/4(to_workspace_enb) -> to_workspace_enable/1
  Write_control_subsys/5(frame_num) -> frame_num/1
  X_init/1 -> Write_control_subsys/5(x_init)
  serialize/1(serial) -> deserialize1/1(serialin), serialized_data/1

== system MOSSE_HDL_final/DSP_Builder_Compute_PSR/Counter ==
  ena : Inport
  sclr : Inport  Port=2
  Comparator1 : allblocks_alteradspbuilder2/Comparator  direction=a == b  pipeline_display=0  allowFloatingPointOverride=on  logOutputs=off  logFile=d:\Project\AutoTracking\model\MOSSE_work\MOSSE_model\MOSSE_Final_models\tb_MOSSE_HDL_final\MOSSE%5FHDL%5Ffinal_DSP%5FBuilder%5FCompute%5FPSR_Counter_Comparator1.fixedpointlog
  Constant : allblocks_alteradspbuilder2/Constant  mask_cst=4095  BusType=Unsigned Integer  bwl=16  bwr=0  roundMode=Truncate  satMode=Wrap  SpecifyClock=off  allowFloatingPointOverride=on  logOutputs=off  logFile=d:\Project\AutoTracking\model\MOSSE_work\MOSSE_model\MOSSE_Final_models\tb_MOSSE_HDL_final\MOSSE%5FHDL%5Ffinal_DSP%5FBuilder%5FCompute%5FPSR_Counter_Constant.fixedpointlog
  Counter : allblocks_alteradspbuilder2/Counter  BusType=Unsigned Integer  bwl=16  bwr=0  use_modulo=on  modulo=4100  SpecifyClock=off  direction=Increment  use_sload=off  use_sset=off  svalue=1  use_clk_ena=off  use_ena=on  use_sclr=on  pipeline_display=1
  finish : Outport
  counter : Outport  Port=2
  wires:
  Constant/1 -> Comparator1/1
  Counter/1 -> counter/1, Comparator1/2
  Comparator1/1 -> finish/1
  sclr/1 -> Counter/2
  ena/1 -> Counter/1

== system MOSSE_HDL_final/DSP_Builder_Compute_PSR/Maximum ==
  finish_flag : Inport
  counter : Inport  Port=2
  Input_data : Inport  Port=3
  max_count_ena : Inport  Port=4
  max_reset : Inport  Port=5
  Comparator : allblocks_alteradspbuilder2/Comparator  direction=a < b  pipeline_display=0  allowFloatingPointOverride=on  logOutputs=off  logFile=d:\Project\AutoTracking\model\MOSSE_work\MOSSE_model\MOSSE_Final_models\tb_MOSSE_HDL_final\MOSSE%5FHDL%5Ffinal_DSP%5FBuilder%5FCompute%5FPSR_Maximum_Comparator.fixedpointlog
  Constant1 : allblocks_alteradspbuilder2/Constant  mask_cst=1  BusType=Single Bit  bwl=24  bwr=0  roundMode=Truncate  satMode=Wrap  SpecifyClock=off  allowFloatingPointOverride=on  logOutputs=off  logFile=d:\Project\AutoTracking\model\MOSSE_work\MOSSE_model\MOSSE_Final_models\tb_MOSSE_HDL_final\MOSSE%5FHDL%5Ffinal_DSP%5FBuilder%5FCompute%5FPSR_Maximum_Constant1.fixedpointlog
  Constant2 : allblocks_alteradspbuilder2/Constant  mask_cst=1  BusType=Single Bit  bwl=24  bwr=0  roundMode=Truncate  satMode=Wrap  SpecifyClock=off  allowFloatingPointOverride=on  logOutputs=off  logFile=d:\Project\AutoTracking\model\MOSSE_work\MOSSE_model\MOSSE_Final_models\tb_MOSSE_HDL_final\MOSSE%5FHDL%5Ffinal_DSP%5FBuilder%5FCompute%5FPSR_Maximum_Constant2.fixedpointlog
  Delay1 : allblocks_alteradspbuilder2/Delay  pipeline=2  pipeline_display=2  ClockPhase=1  use_ena=off  use_sclr=off  allowFloatingPointOverride=on  logOutputs=off  logFile=d:\Project\AutoTracking\model\MOSSE_work\MOSSE_model\MOSSE_Final_models\tb_MOSSE_HDL_final\MOSSE%5FHDL%5Ffinal_DSP%5FBuilder%5FCompute%5FPSR_Maximum_Delay1.fixedpointlog  use_init=off  reset_value=1
  Delay2 : allblocks_alteradspbuilder2/Delay  pipeline=1  pipeline_display=1  ClockPhase=1  use_ena=off  use_sclr=off  allowFloatingPointOverride=on  logOutputs=off  logFile=d:\Project\AutoTracking\model\MOSSE_work\MOSSE_model\MOSSE_Final_models\tb_MOSSE_HDL_final\MOSSE%5FHDL%5Ffinal_DSP%5FBuilder%5FCompute%5FPSR_Maximum_Delay2.fixedpointlog  use_init=off  reset_value=1
  Delay3 : allblocks_alteradspbuilder2/Delay  pipeline=1  pipeline_display=1  ClockPhase=1  use_ena=off  use_sclr=off  allowFloatingPointOverride=on  logOutputs=off  logFile=d:\Project\AutoTracking\model\MOSSE_work\MOSSE_model\MOSSE_Final_models\tb_MOSSE_HDL_final\MOSSE%5FHDL%5Ffinal_DSP%5FBuilder%5FCompute%5FPSR_Maximum_Delay3.fixedpointlog  use_init=off  reset_value=1
  Flipflop : allblocks_alteradspbuilder2/Flipflop  mode=DFFE  BusType=Signed Integer  bwl=16  bwr=2  pipeline_display=1
  Flipflop1 : allblocks_alteradspbuilder2/Flipflop  mode=DFFE  BusType=Signed Integer  bwl=16  bwr=2  pipeline_display=1
  Logical Bit Operator : allblocks_alteradspbuilder2/Logical Bit Operator  LogicalOperator=NOT  user_inputs=2  pipeline_display=0
  Multiplexer : allblocks_alteradspbuilder2/Multiplexer  numInputs=2  pipeline=0  oneHot=off  pipeline_display=0  use_ena=off  use_aclr=off  allowFloatingPointOverride=on  logOutputs=off  logFile=d:\Project\AutoTracking\model\MOSSE_work\MOSSE_model\MOSSE_Final_models\tb_MOSSE_HDL_final\MOSSE%5FHDL%5Ffinal_DSP%5FBuilder%5FCompute%5FPSR_Maximum_Multiplexer.fixedpointlog
  Multiplexer1 : allblocks_alteradspbuilder2/Multiplexer  numInputs=2  pipeline=0  oneHot=off  pipeline_display=0  use_ena=off  use_aclr=off  allowFloatingPointOverride=on  logOutputs=off  logFile=d:\Project\AutoTracking\model\MOSSE_work\MOSSE_model\MOSSE_Final_models\tb_MOSSE_HDL_final\MOSSE%5FHDL%5Ffinal_DSP%5FBuilder%5FCompute%5FPSR_Maximum_Multiplexer1.fixedpointlog
  Multiplexer2 : allblocks_alteradspbuilder2/Multiplexer  numInputs=2  pipeline=0  oneHot=off  pipeline_display=0  use_ena=off  use_aclr=off  allowFloatingPointOverride=on  logOutputs=off  logFile=d:\Project\AutoTracking\model\MOSSE_work\MOSSE_model\MOSSE_Final_models\tb_MOSSE_HDL_final\MOSSE%5FHDL%5Ffinal_DSP%5FBuilder%5FCompute%5FPSR_Maximum_Multiplexer2.fixedpointlog
  max_finish : Outport
  Max_value : Outport  Port=2
  max_num : Outport  Port=3
  delay : Outport  Port=4
  wires:
  Comparator/1 -> Multiplexer/1, Multiplexer1/1
  Flipflop/1 -> Comparator/1, Multiplexer2/3, Multiplexer/2
  Multiplexer/1 -> Flipflop/1
  Constant2/1 -> Flipflop/3, Flipflop/2
  Input_data/1 -> Multiplexer/3, Comparator/2
  Flipflop1/1 -> max_num/1, Multiplexer1/2
  Multiplexer1/1 -> Flipflop1/1
  Constant1/1 -> Flipflop1/3, Flipflop1/2
  counter/1 -> Multiplexer1/3
  Delay1/1 -> max_finish/1, Delay3/1
  max_count_ena/1 -> Multiplexer2/1
  Multiplexer2/1 -> Delay2/1
  Delay2/1 -> Multiplexer2/2, Max_value/1
  Delay3/1 -> delay/1
  finish_flag/1 -> Delay1/1
  Logical Bit Operator/1 -> Flipflop1/4, Flipflop/4
  max_reset/1 -> Logical Bit Operator/1

== system MOSSE_HDL_final/DSP_Builder_Compute_PSR/Mean1 ==
  finish_flag : Inport
  Input_data : Inport  Port=2
  mean_count_ena : Inport  Port=3
  mean_reset : Inport  Port=4
  Barrel Shifter : allblocks_alteradspbuilder2/Barrel Shifter  BusType=Signed Integer  bwl=32  bwr=8  pipeline=off  infer_distance=off  distance_length=4  ShiftDirection=Shift right  use_ena=off  use_aclr=off  UseDedicatedCircuitry=off  pipeline_display=0  allowFloatingPointOverride=on  logOutputs=off  logFile=d:\Project\AutoTracking\model\MOSSE_work\MOSSE_model\MOSSE_Final_models\tb_MOSSE_HDL_final\MOSSE%5FHDL%5Ffinal_DSP%5FBuilder%5FCompute%5FPSR_Mean1_Barrel+Shifter.fixedpointlog
  Constant2 : allblocks_alteradspbuilder2/Constant  mask_cst=12  BusType=Unsigned Integer  bwl=4  bwr=0  roundMode=Truncate  satMode=Wrap  SpecifyClock=off  allowFloatingPointOverride=on  logOutputs=off  logFile=d:\Project\AutoTracking\model\MOSSE_work\MOSSE_model\MOSSE_Final_models\tb_MOSSE_HDL_final\MOSSE%5FHDL%5Ffinal_DSP%5FBuilder%5FCompute%5FPSR_Mean1_Constant2.fixedpointlog
  Delay1 : allblocks_alteradspbuilder2/Delay  pipeline=1  pipeline_display=1  ClockPhase=1  use_ena=off  use_sclr=off  allowFloatingPointOverride=on  logOutputs=off  logFile=d:\Project\AutoTracking\model\MOSSE_work\MOSSE_model\MOSSE_Final_models\tb_MOSSE_HDL_final\MOSSE%5FHDL%5Ffinal_DSP%5FBuilder%5FCompute%5FPSR_Mean1_Delay1.fixedpointlog  use_init=off  reset_value=1
  Delay2 : allblocks_alteradspbuilder2/Delay  pipeline=1  pipeline_display=1  ClockPhase=1  use_ena=off  use_sclr=off  allowFloatingPointOverride=on  logOutputs=off  logFile=d:\Project\AutoTracking\model\MOSSE_work\MOSSE_model\MOSSE_Final_models\tb_MOSSE_HDL_final\MOSSE%5FHDL%5Ffinal_DSP%5FBuilder%5FCompute%5FPSR_Mean1_Delay2.fixedpointlog  use_init=off  reset_value=1
  Multiplexer2 : allblocks_alteradspbuilder2/Multiplexer  numInputs=2  pipeline=0  oneHot=off  pipeline_display=0  use_ena=off  use_aclr=off  allowFloatingPointOverride=on  logOutputs=off  logFile=d:\Project\AutoTracking\model\MOSSE_work\MOSSE_model\MOSSE_Final_models\tb_MOSSE_HDL_final\MOSSE%5FHDL%5Ffinal_DSP%5FBuilder%5FCompute%5FPSR_Mean1_Multiplexer2.fixedpointlog
  Pipelined Adder : allblocks_alteradspbuilder2/Pipelined Adder  BusType=Signed Integer  bwl=32  bwr=0  pipeline=1  pipeline_display=1  AddSubDirection=ADD  use_cin=off  use_ovl=off  use_addsub=off  use_ena=off  use_aclr=on  or_aclr_inputs=off
  mean_finish : Outport
  mean_value : Outport  Port=2
  wires:
  Constant2/1 -> Barrel Shifter/2
  Pipelined Adder/1 -> Pipelined Adder/1, Barrel Shifter/1
  Input_data/1 -> Pipelined Adder/2
  Barrel Shifter/1 -> Multiplexer2/3
  mean_count_ena/1 -> Multiplexer2/1
  Multiplexer2/1 -> Delay2/1
  Delay2/1 -> mean_value/1, Multiplexer2/2
  finish_flag/1 -> Delay1/1
  Delay1/1 -> mean_finish/1
  mean_reset/1 -> Pipelined Adder/3

== system MOSSE_HDL_final/DSP_Builder_Compute_PSR/Psr1 ==
  max : Inport
  mean : Inport  Port=2
  std : Inport  Port=3
  psr_count_ena : Inport  Port=4
  std_finish : Inport  Port=5
  Delay1 : allblocks_alteradspbuilder2/Delay  pipeline=1  pipeline_display=1  ClockPhase=1  use_ena=off  use_sclr=off  allowFloatingPointOverride=on  logOutputs=off  logFile=d:\Project\AutoTracking\model\MOSSE_work\MOSSE_model\MOSSE_Final_models\tb_MOSSE_HDL_final\MOSSE%5FHDL%5Ffinal_DSP%5FBuilder%5FCompute%5FPSR_Psr1_Delay1.fixedpointlog  use_init=off  reset_value=1
  Delay2 : allblocks_alteradspbuilder2/Delay  pipeline=1  pipeline_display=1  ClockPhase=1  use_ena=off  use_sclr=off  allowFloatingPointOverride=on  logOutputs=off  logFile=d:\Project\AutoTracking\model\MOSSE_work\MOSSE_model\MOSSE_Final_models\tb_MOSSE_HDL_final\MOSSE%5FHDL%5Ffinal_DSP%5FBuilder%5FCompute%5FPSR_Psr1_Delay2.fixedpointlog  use_init=off  reset_value=1
  Divider : allblocks_alteradspbuilder2/Divider  BusType=Signed Integer  bwl=32  bwr=0  pipeline=0  pipeline_display=0  use_ena=off  use_aclr=off
  Multiplexer3 : allblocks_alteradspbuilder2/Multiplexer  numInputs=2  pipeline=0  oneHot=off  pipeline_display=0  use_ena=off  use_aclr=off  allowFloatingPointOverride=on  logOutputs=off  logFile=d:\Project\AutoTracking\model\MOSSE_work\MOSSE_model\MOSSE_Final_models\tb_MOSSE_HDL_final\MOSSE%5FHDL%5Ffinal_DSP%5FBuilder%5FCompute%5FPSR_Psr1_Multiplexer3.fixedpointlog
  Pipelined Adder : allblocks_alteradspbuilder2/Pipelined Adder  BusType=Signed Integer  bwl=32  bwr=0  pipeline=0  pipeline_display=0  AddSubDirection=SUB  use_cin=off  use_ovl=off  use_addsub=off  use_ena=off  use_aclr=off  or_aclr_inputs=on
  Psr_finish : Outport
  psr : Outport  Port=2
  wires:
  Pipelined Adder/1 -> Divider/1
  Divider/1 -> Multiplexer3/3
  max/1 -> Pipelined Adder/1
  mean/1 -> Pipelined Adder/2
  std/1 -> Divider/2
  psr_count_ena/1 -> Multiplexer3/1
  Multiplexer3/1 -> Delay2/1
  Delay2/1 -> psr/1, Multiplexer3/2
  std_finish/1 -> Delay1/1
  Delay1/1 -> Psr_finish/1
